simulink model "pitch_rate_controller_tuner"  (R2024b)
settings: Solver=ode1  StartTime=0.0  StopTime=120  FixedStep=0.1  RelTol=1e-3
values from neighbouring files (symbols this model uses):
  A_pitch_rate = [0 0; 1 0]    [main.m]
  B_pitch_rate = [(d_tcg * T_g_full_throttle / I_z); 0]    [main.m]
  C_pitch = [0, 1]    [main.m]
  C_pitch_rate = [1 0]    [main.m]
  D_pitch = 0    [main.m]
  D_pitch_rate = 0    [main.m]
  IC_pitch_ss = [0 theta_0]    [main.m]
  max_rate_rad = deg2rad(max_rate)    [main.m]
libraries: simulink_extras x5, slpidlib x1
settings Model: Creator=jonathanvanzyl  LastModifiedBy=jonathanvanzyl

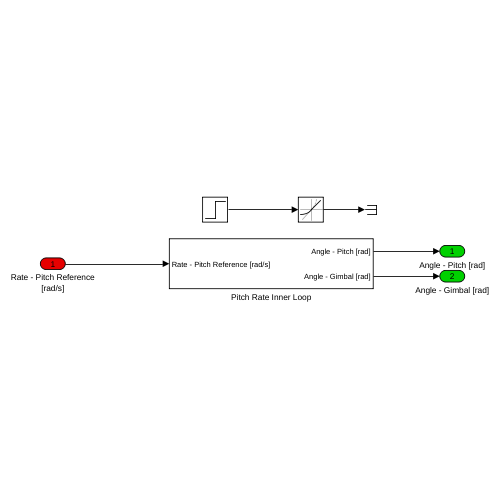
[thumbnail: Simulink's stored preview of the top-level diagram]
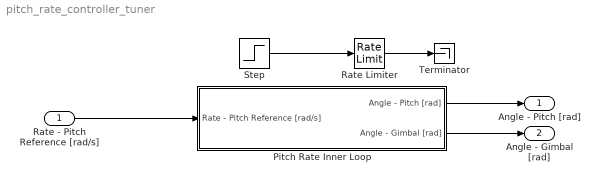
== system pitch_rate_controller_tuner ==
  Rate - Pitch Reference [rad/s] : Inport
  Pitch Rate Inner Loop : Subsystem
  Rate Limiter : RateLimiter  RisingSlewLimit=max_rate_rad*4  FallingSlewLimit=-max_rate_rad  SampleTimeMode=inherited
  Step : Step  SampleTime=0
  Terminator : Terminator
  Angle - Pitch [rad] : Outport
  Angle - Gimbal [rad] : Outport  Port=2
  wires:
  Pitch Rate Inner Loop/1(Angle - Pitch [rad]) -> Angle - Pitch [rad]/1
  Rate - Pitch Reference [rad/s]/1 -> Pitch Rate Inner Loop/1(Rate - Pitch Reference [rad/s])
  Step/1 -> Rate Limiter/1
  Rate Limiter/1 -> Terminator/1
  Pitch Rate Inner Loop/2(Angle - Gimbal [rad]) -> Angle - Gimbal [rad]/1

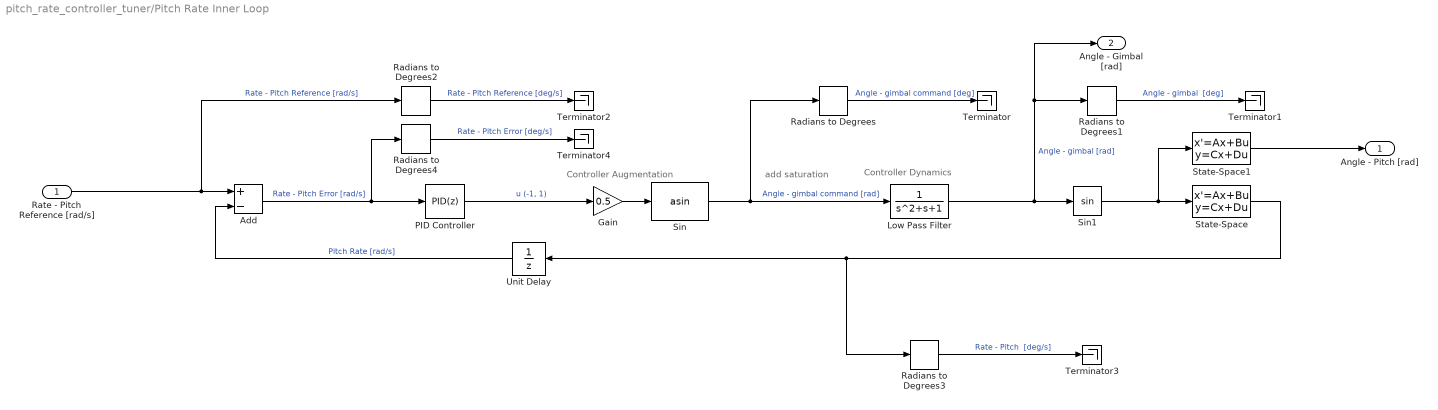
== system pitch_rate_controller_tuner/Pitch Rate Inner Loop ==
  note: Controller Dynamics
  note: Controller Augmentation
  note: add saturation
  Rate - Pitch Reference [rad/s] : Inport
  Add : Sum  Inputs=+-
  Gain : Gain  Gain=0.5
  Low Pass Filter : TransferFcn  Denominator=[1 1 1]
  PID Controller : slpidlib/PID Controller  Controller=PID  Form=Parallel  TimeDomain=Discrete-time  UseExternalTs=off  SampleTime=-1  IntegratorMethod=Forward Euler  FilterMethod=Forward Euler  ControllerParametersSource=internal  P=7.15245081348456  I=0.496256878001195  UseKiTs=off  D=10.5753324079984  UseExternalDerivativeSource=off  N=16.0083835036622  UseFilter=on  TunerSelectOption=Transfer Function Based (PID Tuner App)  InitialConditionSource=internal  InitialConditionForIntegrator=0  InitialConditionForFilter=0  DifferentiatorICPrevScaledInput=0  ExternalReset=none  TrackingMode=off  Kt=1  LimitOutput=off  SatLimitsSource=internal  UpperSaturationLimit=inf  LowerSaturationLimit=-inf  LinearizeAsGain=on  AntiWindupMode=none  Kb=1  LimitIntegrator=off  UpperIntegratorSaturationLimit=inf  LowerIntegratorSaturationLimit=-inf  POutMin=[]  POutMax=[]  IOutMin=[]  IOutMax=[]  DOutMin=[]  DOutMax=[]  NOutMin=[]  NOutMax=[]  SumOutMin=-1  SumOutMax=1  SaturationOutMin=[]  SaturationOutMax=[]  PParamMin=[]  PParamMax=[]  IParamMin=[]  IParamMax=[]  DParamMin=[]  DParamMax=[]  NParamMin=[]  NParamMax=[]  KbParamMin=[]  KbParamMax=[]  KtParamMin=[]  KtParamMax=[]  KbOutMin=[]  KbOutMax=[]  KtOutMin=[]  KtOutMax=[]  IntegratorOutMin=[]  IntegratorOutMax=[]  FilterOutMin=[]  FilterOutMax=[]  SumI1OutMin=[]  SumI1OutMax=[]  SumI2OutMin=[]  SumI2OutMax=[]  SumI3OutMin=[]  SumI3OutMax=[]  SumI4OutMin=[]  SumI4OutMax=[]  SumDOutMin=[]  SumDOutMax=[]  DifferentiatorOutMin=[]  DifferentiatorOutMax=[]  FilterDiffOutCoefMin=[]  FilterDiffOutCoefMax=[]  ReciprocalOutMin=[]  ReciprocalOutMax=[]  SumDenOutMin=[]  SumDenOutMax=[]  SumNumOutMin=[]  SumNumOutMax=[]  DivideOutMin=[]  DivideOutMax=[]  UdiffTsProdOutMin=[]  UdiffTsProdOutMax=[]  NTsProdOutMin=[]  NTsProdOutMax=[]  UintegralTsProdOutMin=[]  UintegralTsProdOutMax=[]  UngainTsProdOutMin=[]  UngainTsProdOutMax=[]  ClampingZeroOutDataTypeStr=Inherit: Inherit via back propagation  ClampingZeroOutMin=[]  ClampingZeroOutMax=[]  FilterDenConstantOutDataTypeStr=Inherit: Inherit via back propagation  FilterDenConstantOutMin=[]  FilterDenConstantOutMax=[]  PCopyOutDataTypeStr=Inherit: Inherit via back propagation  PCopyOutMin=[]  PCopyOutMax=[]  NCopyOutDataTypeStr=Inherit: Inherit via back propagation  NCopyOutMin=[]  NCopyOutMax=[]  IntegratorContinuousStateAttributes=''  IntegratorStateMustResolveToSignalObject=off  IntegratorRTWStateStorageClass=Auto  FilterContinuousStateAttributes=''  FilterStateMustResolveToSignalObject=off  FilterRTWStateStorageClass=Auto  ParallelPVariant=InternalParameters  IdealPVariant=Disabled  IVariant=InternalParameters  DVariant=InternalParameters  IntegratorVariant=Discrete  SatVariant=Disabled  AWVariant=Passthrough  PCopyVariant=Disabled  TRVariant=Disabled  FdbkBlocksVariant=Forward  IdealPFdbkVariant=Disabled  SatFdbkVariant=Disabled  DerivativeFilterVariant=ForwardEulerFilter  NVariant=InternalParameters  NCopyVariant=Disabled  FilterICVariant=InternalICsFilter  IntegratorICVariant=InternalICs  ExternalResetVariant=Disabled  TRSumVariant=Passthrough  SumFdbkVariant=Disabled  SumVariant=Sum_PID  TsampFilterVariant=InternalTs  TsampNgainVariant=Passthrough  TsampIntegralVariant=Disabled_SignalSpec  ExternalSaturationOutDataTypeStr=Inherit: Same as second input  DerivativeSourceVariant=ErrorSignal  PreIntVariant=InternalPreInt
  Radians to Degrees{,1..4} (5 alike) : simulink_extras/Transformations/Radians to Degrees
  Sin : Trigonometry  Operator=asin
  Sin1 : Trigonometry
  State-Space : StateSpace  A=A_pitch_rate  B=B_pitch_rate  C=C_pitch_rate  D=D_pitch_rate  InitialCondition=IC_pitch_ss
  State-Space1 : StateSpace  A=A_pitch_rate  B=B_pitch_rate  C=C_pitch  D=D_pitch  InitialCondition=IC_pitch_ss
  Terminator{,1..4} (5 alike) : Terminator
  Unit Delay : UnitDelay  SampleTime=-1  HasFrameUpgradeWarning=on
  Angle - Pitch [rad] : Outport
  Angle - Gimbal [rad] : Outport  Port=2
  wires:
  Low Pass Filter/1 -> Angle - Gimbal [rad]/1, Radians to Degrees1/1, Sin1/1  "Angle - gimbal [rad]"
  Radians to Degrees4/1 -> Terminator4/1  "Rate - Pitch Error [deg/s]"
  PID Controller/1 -> Gain/1  "u (-1, 1)"
  Sin1/1 -> State-Space1/1, State-Space/1
  Radians to Degrees3/1 -> Terminator3/1  "Rate - Pitch  [deg/s]"
  Gain/1 -> Sin/1
  Rate - Pitch Reference [rad/s]/1 -> Radians to Degrees2/1, Add/1  "Rate - Pitch Reference [rad/s]"
  Radians to Degrees2/1 -> Terminator2/1  "Rate - Pitch Reference [deg/s]"
  Add/1 -> Radians to Degrees4/1, PID Controller/1  "Rate - Pitch Error [rad/s]"
  Unit Delay/1 -> Add/2  "Pitch Rate [rad/s]"
  Sin/1 -> Radians to Degrees/1, Low Pass Filter/1  "Angle - gimbal command [rad]"
  Radians to Degrees/1 -> Terminator/1  "Angle - gimbal command [deg]"
  Radians to Degrees1/1 -> Terminator1/1  "Angle - gimbal  [deg]"
  State-Space/1 -> Radians to Degrees3/1, Unit Delay/1
  State-Space1/1 -> Angle - Pitch [rad]/1
